simulink model "Project_NoControl"  (R2021b)
settings: Solver=VariableStepAuto  StartTime=0.0  StopTime=tt_end  RelTol=1e-3
values from neighbouring files (symbols this model uses):
  h2 = 0.12    [RPR_Simscape.m]    (also in RPR_Simulation.m = figure(2); RPR_kin_dyn_q.m = figure(2); RPR_kin_dyn_s.m = figure(2); plotRPR.m = triad('Parent',axs,'Scale',0.05,'LineWidth',0.5,'Tag','','Ma)
  h3 = 0.12    [RPR_Simscape.m]    (also in RPR_Simulation.m = figure(3); RPR_kin_dyn_q.m = figure(3); RPR_kin_dyn_s.m = figure(3); plotRPR.m = triad('Parent',axs,'Scale',0.05,'LineWidth',0.5,'Tag','','Ma)
  l2 = L(2)    [M_matrix.m]    (also in RPR_Simscape.m = 0.3; RPR_Simulation.m = 0.3; RPR_dir.m; RPR_dir_ext.m)
  l3 = L(3)    [M_matrix.m]    (also in RPR_Simscape.m = 0.5; RPR_Simulation.m = 0.5; RPR_dir.m; RPR_dir_ext.m)
  l4 = 0.65    [RPR_Simscape.m]    (also in RPR_Simulation.m = 0.6; RPR_dir_ext.m = L(4); RPR_inv.m = L(4); RPR_jac_ext.m = L(4))
  l5 = L(5)    [M_matrix.m]    (also in RPR_Simscape.m = 0.5; RPR_Simulation.m = 0.5; RPR_dir.m; RPR_dir_ext.m)
  m = [m1,m2,m3,m4,m5,mg]    [RPR_Simulation.m]    (also in RPR_kin_dyn_q.m; RPR_kin_dyn_q_multiple.m = [m1,m2,m3,m4,m5]; RPR_kin_dyn_s.m = [m1,m2,m3,m4,m5]; RPR_kin_dyn_s_multiple.m = [m1,m2,m3,m4,m5])
  s = [x(i) y(i) z(i)]'    [RPR_Simulation.m]    (also in RPR_dir.m = zeros(3,1); RPR_kin_dyn_q.m = RPR_dir([q1(i),q2(i),q3(i)],Length); RPR_kin_dyn_q_multiple.m = RPR_dir([q1(i),q2(i),q3(i)],Length); RPR_kin_dyn_s.m)
  w2 = 0.12    [RPR_Simscape.m]
  w3 = 0.12    [RPR_Simscape.m]
undefined symbols (not defined in the file or in its folder): sigbuilder_block, X, Y, Z
libraries: sm_lib x27, nesl_utility x25
(part 2 of 2)

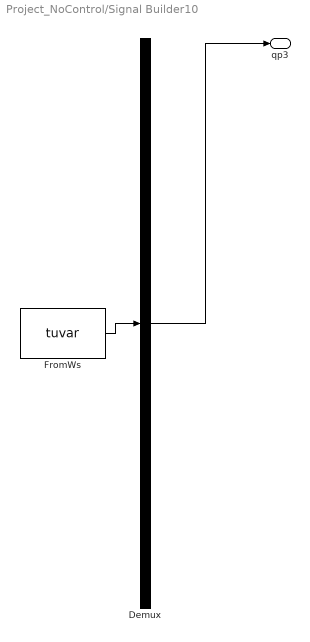
== system Project_NoControl/Signal Builder10 ==
  Demux : Demux  Tag=STV Demux  Outputs=1
      settings: DisplayOption=none
  FromWs : FromWorkspace  Tag=STV FromWs  VariableName=tuvar
      SigBuilderData=|
      | common.afterFinalStr = 'Extrapolate'
      | common.sampleTime = 0
      | dataSet.timeRange = [0 8.72479475862]
      | dataSet.name = 'Joint 3'
      | sbobj.Groups.Name = 'Joint 3'
      | sbobj.Groups.Signals.Name = 'qp3'
      | sbobj.Groups.Signals.XData = [0 0.00229093367015 0.00458186734029 0.00687280101044 0.00916373468059 0.0114546683507 0.0137456020209 0.016036535691 0.0183274693612 0.0206184030313 0.0229093367015 0.0252002703716 ... (4450 elements, 1x4450)]
      | sbobj.Groups.Signals.YData = [0 0.00287062590972 0.00574125181944 0.00861187772916 0.0114825036389 0.0143531295486 0.0172237554583 0.020094381368 0.0229650072778 0.0258356331875 0.0287062590972 0.0315768850069 ... (4450 elements, 1x4450)]
      | sbobj.Groups.TimeRange = [0 8.72479475862]
  qp3 : Outport  Tag=STV Outport
  wires:
  Demux/1 -> qp3/1
  FromWs/1 -> Demux/1

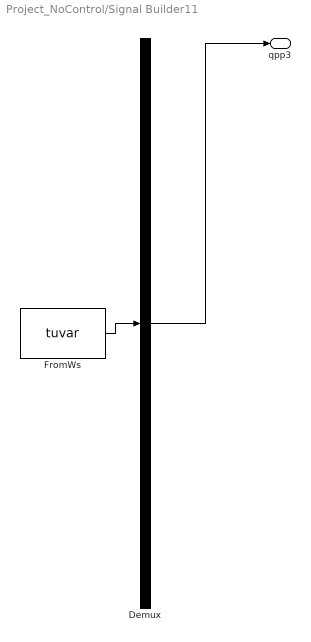
== system Project_NoControl/Signal Builder11 ==
  Demux : Demux  Tag=STV Demux  Outputs=1
      settings: DisplayOption=none
  FromWs : FromWorkspace  Tag=STV FromWs  VariableName=tuvar
      SigBuilderData=|
      | common.afterFinalStr = 'Extrapolate'
      | common.sampleTime = 0
      | dataSet.timeRange = [0 8.72479475862]
      | dataSet.name = 'Joint 3'
      | sbobj.Groups.Name = 'Joint 3'
      | sbobj.Groups.Signals.Name = 'qpp3'
      | sbobj.Groups.Signals.XData = [0 0.00229093367015 0.00458186734029 0.00687280101044 0.00916373468059 0.0114546683507 0.0137456020209 0.016036535691 0.0183274693612 0.0206184030313 0.0229093367015 0.0252002703716 ... (4450 elements, 1x4450)]
      | sbobj.Groups.Signals.YData = [1.25303754846 1.25303754846 1.25303754846 1.25303754846 1.25303754846 1.25303754846 1.25303754846 1.25303754846 1.25303754846 1.25303754846 1.25303754846 1.25303754846 ... (4450 elements, 1x4450)]
      | sbobj.Groups.TimeRange = [0 8.72479475862]
  qpp3 : Outport  Tag=STV Outport
  wires:
  FromWs/1 -> Demux/1
  Demux/1 -> qpp3/1

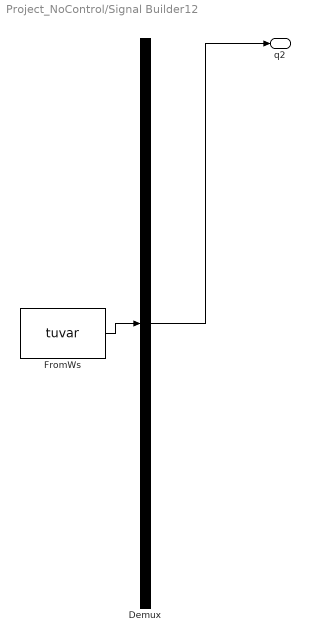
== system Project_NoControl/Signal Builder12 ==
  Demux : Demux  Tag=STV Demux  Outputs=1
      settings: DisplayOption=none
  FromWs : FromWorkspace  Tag=STV FromWs  VariableName=tuvar
      SigBuilderData=|
      | common.afterFinalStr = 'Extrapolate'
      | common.sampleTime = 0
      | dataSet.timeRange = [0 8.72479475862]
      | dataSet.name = 'Joint 2'
      | sbobj.Groups.Name = 'Joint 2'
      | sbobj.Groups.Signals.Name = 'q2'
      | sbobj.Groups.Signals.XData = [0 0.00229093367015 0.00458186734029 0.00687280101044 0.00916373468059 0.0114546683507 0.0137456020209 0.016036535691 0.0183274693612 0.0206184030313 0.0229093367015 0.0252002703716 ... (4450 elements, 1x4450)]
      | sbobj.Groups.Signals.YData = [0.1 0.100002598626 0.100010394504 0.100023387634 0.100041578017 0.100064965651 0.100093550537 0.100127332676 0.100166312067 0.100210488709 0.100259862604 0.100314433751 ... (4450 elements, 1x4450)]
      | sbobj.Groups.TimeRange = [0 8.72479475862]
  q2 : Outport  Tag=STV Outport
  wires:
  Demux/1 -> q2/1
  FromWs/1 -> Demux/1

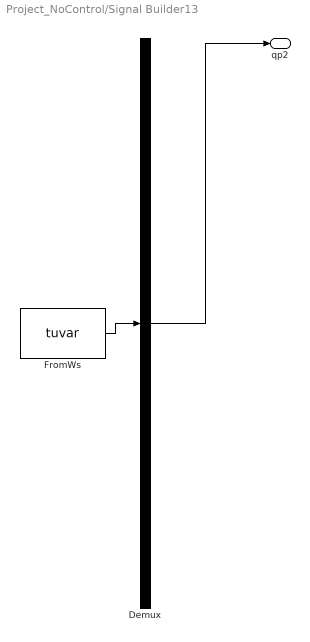
== system Project_NoControl/Signal Builder13 ==
  Demux : Demux  Tag=STV Demux  Outputs=1
      settings: DisplayOption=none
  FromWs : FromWorkspace  Tag=STV FromWs  VariableName=tuvar
      SigBuilderData=|
      | common.afterFinalStr = 'Extrapolate'
      | common.sampleTime = 0
      | dataSet.timeRange = [0 8.72479475862]
      | dataSet.name = 'Joint 2'
      | sbobj.Groups.Name = 'Joint 2'
      | sbobj.Groups.Signals.Name = 'qp2'
      | sbobj.Groups.Signals.XData = [0 0.00229093367015 0.00458186734029 0.00687280101044 0.00916373468059 0.0114546683507 0.0137456020209 0.016036535691 0.0183274693612 0.0206184030313 0.0229093367015 0.0252002703716 ... (4450 elements, 1x4450)]
      | sbobj.Groups.Signals.YData = [0 0.00226861744045 0.00453723488091 0.00680585232136 0.00907446976182 0.0113430872023 0.0136117046427 0.0158803220832 0.0181489395236 0.0204175569641 0.0226861744045 0.024954791845 ... (4450 elements, 1x4450)]
      | sbobj.Groups.TimeRange = [0 8.72479475862]
  qp2 : Outport  Tag=STV Outport
  wires:
  FromWs/1 -> Demux/1
  Demux/1 -> qp2/1

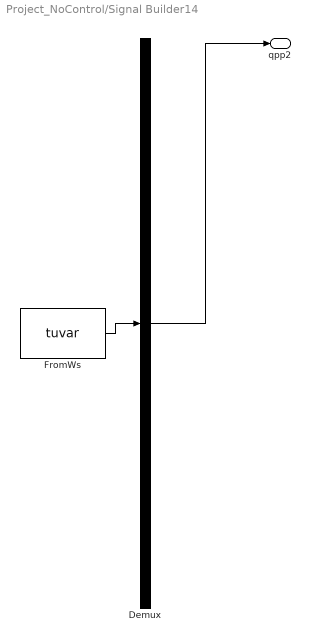
== system Project_NoControl/Signal Builder14 ==
  Demux : Demux  Tag=STV Demux  Outputs=1
      settings: DisplayOption=none
  FromWs : FromWorkspace  Tag=STV FromWs  VariableName=tuvar
      SigBuilderData=|
      | common.afterFinalStr = 'Extrapolate'
      | common.sampleTime = 0
      | dataSet.timeRange = [0 8.72479475862]
      | dataSet.name = 'Joint 2'
      | sbobj.Groups.Name = 'Joint 2'
      | sbobj.Groups.Signals.Name = 'qpp2'
      | sbobj.Groups.Signals.XData = [0 0.00229093367015 0.00458186734029 0.00687280101044 0.00916373468059 0.0114546683507 0.0137456020209 0.016036535691 0.0183274693612 0.0206184030313 0.0229093367015 0.0252002703716 ... (4450 elements, 1x4450)]
      | sbobj.Groups.Signals.YData = [0.990258893139 0.990258893139 0.990258893139 0.990258893139 0.990258893139 0.990258893139 0.990258893139 0.990258893139 0.990258893139 0.990258893139 0.990258893139 0.990258893139 ... (4450 elements, 1x4450)]
      | sbobj.Groups.TimeRange = [0 8.72479475862]
  qpp2 : Outport  Tag=STV Outport
  wires:
  Demux/1 -> qpp2/1
  FromWs/1 -> Demux/1

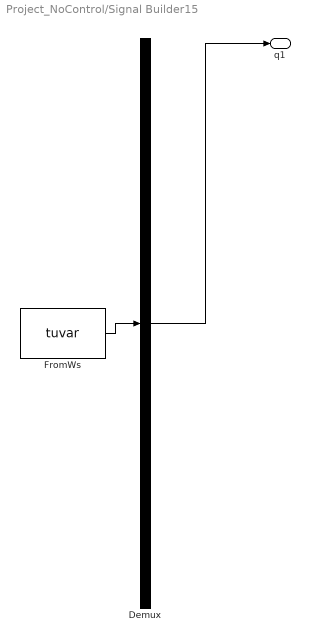
== system Project_NoControl/Signal Builder15 ==
  Demux : Demux  Tag=STV Demux  Outputs=1
      settings: DisplayOption=none
  FromWs : FromWorkspace  Tag=STV FromWs  VariableName=tuvar
      SigBuilderData=|
      | common.afterFinalStr = 'Extrapolate'
      | common.sampleTime = 0
      | dataSet.timeRange = [0 8.72479475862]
      | dataSet.name = 'Joint 1'
      | sbobj.Groups.Name = 'Joint 1'
      | sbobj.Groups.Signals.Name = 'q1'
      | sbobj.Groups.Signals.XData = [0 0.00229093367015 0.00458186734029 0.00687280101044 0.00916373468059 0.0114546683507 0.0137456020209 0.016036535691 0.0183274693612 0.0206184030313 0.0229093367015 0.0252002703716 ... (4450 elements, 1x4450)]
      | sbobj.Groups.Signals.YData = [0 -3.93628281059e-06 -1.57451312432e-05 -3.54265452969e-05 -6.29805249721e-05 -9.8407070269e-05 -0.000141706181187 -0.000192877857727 -0.000251922099888 -0.000318838907671 -0.000393628281076 -0.000476290220102 ... (4450 elements, 1x4450)]
      | sbobj.Groups.TimeRange = [0 8.72479475862]
  q1 : Outport  Tag=STV Outport
  wires:
  FromWs/1 -> Demux/1
  Demux/1 -> q1/1

== system Project_NoControl/Signal Builder16 ==
  Demux : Demux  Tag=STV Demux  Outputs=1
      settings: DisplayOption=none
  FromWs : FromWorkspace  Tag=STV FromWs  VariableName=tuvar
      SigBuilderData=|
      | common.afterFinalStr = 'Extrapolate'
      | common.sampleTime = 0
      | dataSet.timeRange = [0 8.72479475862]
      | dataSet.name = 'Joint 1'
      | sbobj.Groups.Name = 'Joint 1'
      | sbobj.Groups.Signals.Name = 'qp1'
      | sbobj.Groups.Signals.XData = [0 0.00229093367015 0.00458186734029 0.00687280101044 0.00916373468059 0.0114546683507 0.0137456020209 0.016036535691 0.0183274693612 0.0206184030313 0.0229093367015 0.0252002703716 ... (4450 elements, 1x4450)]
      | sbobj.Groups.Signals.YData = [0 -0.00343640050522 -0.00687280101044 -0.0103092015157 -0.0137456020209 -0.0171820025261 -0.0206184030313 -0.0240548035365 -0.0274912040418 -0.030927604547 -0.0343640050522 -0.0378004055574 ... (4450 elements, 1x4450)]
      | sbobj.Groups.TimeRange = [0 8.72479475862]
  qp1 : Outport  Tag=STV Outport
  wires:
  Demux/1 -> qp1/1
  FromWs/1 -> Demux/1

== system Project_NoControl/Signal Builder17 ==
  Demux : Demux  Tag=STV Demux  Outputs=1
      settings: DisplayOption=none
  FromWs : FromWorkspace  Tag=STV FromWs  VariableName=tuvar
      SigBuilderData=|
      | common.afterFinalStr = 'Extrapolate'
      | common.sampleTime = 0
      | dataSet.timeRange = [0 8.72479475862]
      | dataSet.name = 'Joint 1'
      | sbobj.Groups.Name = 'Joint 1'
      | sbobj.Groups.Signals.Name = 'qpp1'
      | sbobj.Groups.Signals.XData = [0 0.00229093367015 0.00458186734029 0.00687280101044 0.00916373468059 0.0114546683507 0.0137456020209 0.016036535691 0.0183274693612 0.0206184030313 0.0229093367015 0.0252002703716 ... (4450 elements, 1x4450)]
      | sbobj.Groups.Signals.YData = [-1.5 -1.5 -1.5 -1.5 -1.5 -1.5 -1.5 -1.5 -1.5 -1.5 -1.5 -1.5 ... (4450 elements, 1x4450)]
      | sbobj.Groups.TimeRange = [0 8.72479475862]
  qpp1 : Outport  Tag=STV Outport
  wires:
  FromWs/1 -> Demux/1
  Demux/1 -> qpp1/1

== system Project_NoControl/Signal Builder9 ==
  Demux : Demux  Tag=STV Demux  Outputs=1
      settings: DisplayOption=none
  FromWs : FromWorkspace  Tag=STV FromWs  VariableName=tuvar
      SigBuilderData=|
      | common.afterFinalStr = 'Extrapolate'
      | common.sampleTime = 0
      | dataSet.timeRange = [0 8.72479475862]
      | dataSet.name = 'Joint 3'
      | sbobj.Groups.Name = 'Joint 3'
      | sbobj.Groups.Signals.Name = 'q3'
      | sbobj.Groups.Signals.XData = [0 0.00229093367015 0.00458186734029 0.00687280101044 0.00916373468059 0.0114546683507 0.0137456020209 0.016036535691 0.0183274693612 0.0206184030313 0.0229093367015 0.0252002703716 ... (4450 elements, 1x4450)]
      | sbobj.Groups.Signals.YData = [0 3.28820677554e-06 1.31528271021e-05 2.95938609794e-05 5.26113084079e-05 8.22051693872e-05 0.000118375443918 0.000161122131999 0.000210445233631 0.000266344748815 0.000328820677549 0.000397873019834 ... (4450 elements, 1x4450)]
      | sbobj.Groups.TimeRange = [0 8.72479475862]
  q3 : Outport  Tag=STV Outport
  wires:
  FromWs/1 -> Demux/1
  Demux/1 -> q3/1
